simulink model "lab1_without_fuzzy_001"  (R2016a)
settings: Solver=ode45  StartTime=0.0  StopTime=10  RelTol=1e-3
values from neighbouring files (symbols this model uses):
  FORCE_Range_1 = -150    [fuzzy_controller_3_trimf_params.m]    (also in fuzzy_controller_5_gauss_params.m; fuzzy_controller_5_gbell_params.m; fuzzy_controller_5_trimf_optimal_params.m; fuzzy_controller_5_trimf_params.m)
  FORCE_Range_2 = 150    [fuzzy_controller_3_trimf_params.m]    (also in fuzzy_controller_5_gauss_params.m; fuzzy_controller_5_gbell_params.m; fuzzy_controller_5_trimf_optimal_params.m; fuzzy_controller_5_trimf_params.m)
  g = 9.81    [Variables_001.m]
  Kd = 141    [Variables_001.m]
  Kp = 1108    [Variables_001.m]
  l = 1    [Variables_001.m]
  M = 10    [Variables_001.m]
  m = 1    [Variables_001.m]
  q0 = 0.1    [Variables_001.m]
  taum = 0.001    [Variables_001.m]
undefined symbols (not defined in the file): fi_1_a, fi_1_b, fi_1_c, fi_1_d, fi_2_a, fi_2_b, fi_2_c, fi_3_a, fi_3_b, fi_3_c, fi_4_a, fi_4_b, fi_4_c, fi_5_a, fi_5_b, fi_5_c, fi_5_d, FORCE_1_a, FORCE_1_b, FORCE_1_c, FORCE_2_a, FORCE_2_b, FORCE_2_c, FORCE_3_a, FORCE_3_b, FORCE_3_c, FORCE_4_a, FORCE_4_b, FORCE_4_c, FORCE_5_a, FORCE_5_b, FORCE_5_c, omega_1_a, omega_1_b, omega_1_c, omega_1_d, omega_2_a, omega_2_b, omega_2_c, omega_3_a, omega_3_b, omega_3_c, omega_4_a, omega_4_b, omega_4_c, omega_5_a, omega_5_b, omega_5_c, omega_5_d
libraries: fuzblock x41, fuzwiz x2
(part 2 of 2)

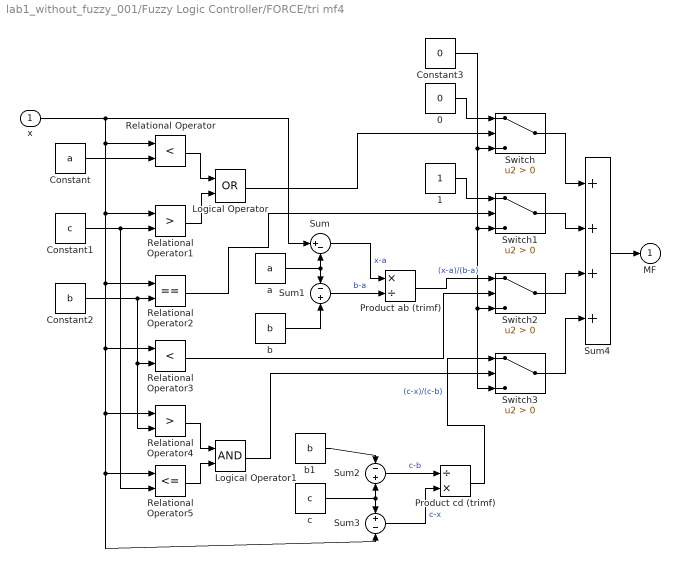
== system lab1_without_fuzzy_001/Fuzzy Logic Controller/FORCE/tri mf4 ==
  x : Inport
  0 : Constant  Value=0
  1 : Constant
  Constant : Constant  Value=a
  Constant1 : Constant  Value=c
  Constant2 : Constant  Value=b
  Constant3 : Constant  Value=0
  Logical Operator : Logic  Operator=OR  AllPortsSameDT=off  OutDataTypeStr=boolean
  Logical Operator1 : Logic  AllPortsSameDT=off  OutDataTypeStr=boolean
  Product ab (trimf) : Product  Inputs=*/  SaturateOnIntegerOverflow=on  InputSameDT=on  OutDataTypeStr=Inherit: Same as first input
  Product cd (trimf) : Product  Inputs=/*  SaturateOnIntegerOverflow=on  InputSameDT=on  OutDataTypeStr=Inherit: Same as first input
  Relational Operator : RelationalOperator  Operator=<  OutDataTypeStr=boolean
  Relational Operator1 : RelationalOperator  Operator=>  OutDataTypeStr=boolean
  Relational Operator2 : RelationalOperator  Operator===  OutDataTypeStr=boolean
  Relational Operator3 : RelationalOperator  Operator=<  OutDataTypeStr=boolean
  Relational Operator4 : RelationalOperator  Operator=>  OutDataTypeStr=boolean
  Relational Operator5 : RelationalOperator  Operator=<=  OutDataTypeStr=boolean
  Sum : Sum  Inputs=|+-  SaturateOnIntegerOverflow=on  InputSameDT=on  OutDataTypeStr=Inherit: Same as first input
  Sum1 : Sum  Inputs=-+  SaturateOnIntegerOverflow=on  InputSameDT=on  OutDataTypeStr=Inherit: Same as first input
  Sum2 : Sum  Inputs=-+  SaturateOnIntegerOverflow=on  InputSameDT=on  OutDataTypeStr=Inherit: Same as first input
  Sum3 : Sum  Inputs=+-  SaturateOnIntegerOverflow=on  InputSameDT=on  OutDataTypeStr=Inherit: Same as first input
  Sum4 : Sum  Inputs=++++
  Switch{,1..3} (4 alike) : Switch  Criteria=u2 > Threshold
  a : Constant  Value=a
  b : Constant  Value=b
  b1 : Constant  Value=b
  c : Constant  Value=c
  MF : Outport
  wires:
  0/1 -> Switch/1
  1/1 -> Switch1/1
  Constant/1 -> Relational Operator/2
  Relational Operator/1 -> Logical Operator/1
  Constant1/1 -> Relational Operator5/2, Relational Operator1/2
  Relational Operator1/1 -> Logical Operator/2
  Product ab (trimf)/1 -> Switch2/1  "(x-a)/(b-a)"
  a/1 -> Sum/2, Sum1/1
  b/1 -> Sum1/2
  Sum/1 -> Product ab (trimf)/1  "x-a"
  Sum1/1 -> Product ab (trimf)/2  "b-a"
  b1/1 -> Sum2/1
  x/1 -> Sum/1, Sum3/2, Relational Operator5/1, Relational Operator4/1, Relational Operator3/1, Relational Operator2/1, Relational Operator1/1, Relational Operator/1
  c/1 -> Sum3/1, Sum2/2
  Sum3/1 -> Product cd (trimf)/2  "c-x"
  Sum2/1 -> Product cd (trimf)/1  "c-b"
  Product cd (trimf)/1 -> Switch3/1  "(c-x)/(c-b)"
  Constant2/1 -> Relational Operator2/2, Relational Operator3/2, Relational Operator4/2
  Relational Operator4/1 -> Logical Operator1/1
  Relational Operator5/1 -> Logical Operator1/2
  Switch/1 -> Sum4/1
  Switch1/1 -> Sum4/2
  Switch2/1 -> Sum4/3
  Switch3/1 -> Sum4/4
  Constant3/1 -> Switch3/3, Switch2/3, Switch1/3, Switch/3
  Logical Operator1/1 -> Switch3/2
  Relational Operator3/1 -> Switch2/2
  Relational Operator2/1 -> Switch1/2
  Logical Operator/1 -> Switch/2
  Sum4/1 -> MF/1

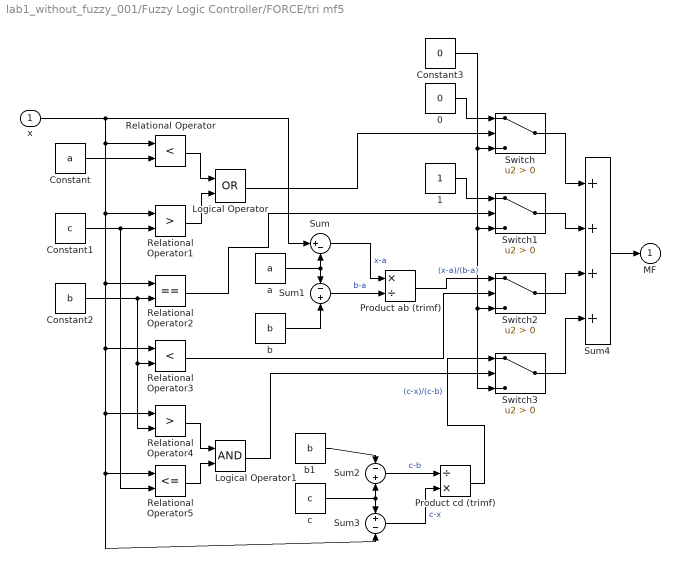
== system lab1_without_fuzzy_001/Fuzzy Logic Controller/FORCE/tri mf5 ==
  x : Inport
  0 : Constant  Value=0
  1 : Constant
  Constant : Constant  Value=a
  Constant1 : Constant  Value=c
  Constant2 : Constant  Value=b
  Constant3 : Constant  Value=0
  Logical Operator : Logic  Operator=OR  AllPortsSameDT=off  OutDataTypeStr=boolean
  Logical Operator1 : Logic  AllPortsSameDT=off  OutDataTypeStr=boolean
  Product ab (trimf) : Product  Inputs=*/  SaturateOnIntegerOverflow=on  InputSameDT=on  OutDataTypeStr=Inherit: Same as first input
  Product cd (trimf) : Product  Inputs=/*  SaturateOnIntegerOverflow=on  InputSameDT=on  OutDataTypeStr=Inherit: Same as first input
  Relational Operator : RelationalOperator  Operator=<  OutDataTypeStr=boolean
  Relational Operator1 : RelationalOperator  Operator=>  OutDataTypeStr=boolean
  Relational Operator2 : RelationalOperator  Operator===  OutDataTypeStr=boolean
  Relational Operator3 : RelationalOperator  Operator=<  OutDataTypeStr=boolean
  Relational Operator4 : RelationalOperator  Operator=>  OutDataTypeStr=boolean
  Relational Operator5 : RelationalOperator  Operator=<=  OutDataTypeStr=boolean
  Sum : Sum  Inputs=|+-  SaturateOnIntegerOverflow=on  InputSameDT=on  OutDataTypeStr=Inherit: Same as first input
  Sum1 : Sum  Inputs=-+  SaturateOnIntegerOverflow=on  InputSameDT=on  OutDataTypeStr=Inherit: Same as first input
  Sum2 : Sum  Inputs=-+  SaturateOnIntegerOverflow=on  InputSameDT=on  OutDataTypeStr=Inherit: Same as first input
  Sum3 : Sum  Inputs=+-  SaturateOnIntegerOverflow=on  InputSameDT=on  OutDataTypeStr=Inherit: Same as first input
  Sum4 : Sum  Inputs=++++
  Switch{,1..3} (4 alike) : Switch  Criteria=u2 > Threshold
  a : Constant  Value=a
  b : Constant  Value=b
  b1 : Constant  Value=b
  c : Constant  Value=c
  MF : Outport
  wires:
  0/1 -> Switch/1
  1/1 -> Switch1/1
  Constant/1 -> Relational Operator/2
  Relational Operator/1 -> Logical Operator/1
  Constant1/1 -> Relational Operator5/2, Relational Operator1/2
  Relational Operator1/1 -> Logical Operator/2
  Product ab (trimf)/1 -> Switch2/1  "(x-a)/(b-a)"
  a/1 -> Sum/2, Sum1/1
  b/1 -> Sum1/2
  Sum/1 -> Product ab (trimf)/1  "x-a"
  Sum1/1 -> Product ab (trimf)/2  "b-a"
  b1/1 -> Sum2/1
  x/1 -> Sum/1, Sum3/2, Relational Operator5/1, Relational Operator4/1, Relational Operator3/1, Relational Operator2/1, Relational Operator1/1, Relational Operator/1
  c/1 -> Sum3/1, Sum2/2
  Sum3/1 -> Product cd (trimf)/2  "c-x"
  Sum2/1 -> Product cd (trimf)/1  "c-b"
  Product cd (trimf)/1 -> Switch3/1  "(c-x)/(c-b)"
  Constant2/1 -> Relational Operator2/2, Relational Operator3/2, Relational Operator4/2
  Relational Operator4/1 -> Logical Operator1/1
  Relational Operator5/1 -> Logical Operator1/2
  Switch/1 -> Sum4/1
  Switch1/1 -> Sum4/2
  Switch2/1 -> Sum4/3
  Switch3/1 -> Sum4/4
  Constant3/1 -> Switch3/3, Switch2/3, Switch1/3, Switch/3
  Logical Operator1/1 -> Switch3/2
  Relational Operator3/1 -> Switch2/2
  Relational Operator2/1 -> Switch1/2
  Logical Operator/1 -> Switch/2
  Sum4/1 -> MF/1

== system lab1_without_fuzzy_001/Fuzzy Logic Controller/fi/trap mf1 ==
  x : Inport
  If Action Subsystem : fuzblock/Membership  Functions/Triangular MF/If Action Subsystem
  If Action Subsystem1 : fuzblock/Membership  Functions/Triangular MF/If Action Subsystem1
  If Action Subsystem2 : fuzblock/Membership  Functions/Trapezoidal MF/If Action Subsystem1
  If Action Subsystem8 : fuzblock/Membership  Functions/Trapezoidal MF/If Action Subsystem3
  If2 : If  IfExpression=(u1 < a) | (u1>d)  ElseIfExpressions=(u1 >= b) & (u1 <= c), u1 < b  ZeroCross=off
  Merge : Merge  Inputs=4
  MF : Outport
  wires:
  If Action Subsystem2/1 -> Merge/3
  If2/3 -> If Action Subsystem2/Action
  If Action Subsystem8/1 -> Merge/4
  If2/4 -> If Action Subsystem8/Action
  If Action Subsystem1/1 -> Merge/2
  If2/2 -> If Action Subsystem1/Action
  If Action Subsystem/1 -> Merge/1
  Merge/1 -> MF/1
  If2/1 -> If Action Subsystem/Action
  x/1 -> If Action Subsystem2/1, If Action Subsystem8/1, If2/1

== system lab1_without_fuzzy_001/Fuzzy Logic Controller/fi/trap mf5 ==
  x : Inport
  If Action Subsystem : fuzblock/Membership  Functions/Triangular MF/If Action Subsystem
  If Action Subsystem1 : fuzblock/Membership  Functions/Triangular MF/If Action Subsystem1
  If Action Subsystem2 : fuzblock/Membership  Functions/Trapezoidal MF/If Action Subsystem1
  If Action Subsystem8 : fuzblock/Membership  Functions/Trapezoidal MF/If Action Subsystem3
  If2 : If  IfExpression=(u1 < a) | (u1>d)  ElseIfExpressions=(u1 >= b) & (u1 <= c), u1 < b  ZeroCross=off
  Merge : Merge  Inputs=4
  MF : Outport
  wires:
  If Action Subsystem2/1 -> Merge/3
  If2/3 -> If Action Subsystem2/Action
  If Action Subsystem8/1 -> Merge/4
  If2/4 -> If Action Subsystem8/Action
  If Action Subsystem1/1 -> Merge/2
  If2/2 -> If Action Subsystem1/Action
  If Action Subsystem/1 -> Merge/1
  Merge/1 -> MF/1
  If2/1 -> If Action Subsystem/Action
  x/1 -> If Action Subsystem2/1, If Action Subsystem8/1, If2/1

== system lab1_without_fuzzy_001/Fuzzy Logic Controller/fi/tri mf2 ==
  x : Inport
  If : If  IfExpression=(u1<a) | (u1>c)  ElseIfExpressions=u1==b, u1 < b  ZeroCross=off
  If Action Subsystem : fuzblock/Membership  Functions/Triangular MF/If Action Subsystem
  If Action Subsystem1 : fuzblock/Membership  Functions/Triangular MF/If Action Subsystem1
  If Action Subsystem2 : fuzblock/Membership  Functions/Triangular MF/If Action Subsystem2
  If Action Subsystem3 : fuzblock/Membership  Functions/Triangular MF/If Action Subsystem3
  Merge : Merge  Inputs=4
  MF : Outport
  wires:
  If Action Subsystem3/1 -> Merge/3
  If/3 -> If Action Subsystem3/Action
  If Action Subsystem2/1 -> Merge/4
  If/4 -> If Action Subsystem2/Action
  If Action Subsystem1/1 -> Merge/2
  If/2 -> If Action Subsystem1/Action
  If Action Subsystem/1 -> Merge/1
  Merge/1 -> MF/1
  If/1 -> If Action Subsystem/Action
  x/1 -> If Action Subsystem3/1, If Action Subsystem2/1, If/1

== system lab1_without_fuzzy_001/Fuzzy Logic Controller/fi/tri mf3 ==
  x : Inport
  If : If  IfExpression=(u1<a) | (u1>c)  ElseIfExpressions=u1==b, u1 < b  ZeroCross=off
  If Action Subsystem : fuzblock/Membership  Functions/Triangular MF/If Action Subsystem
  If Action Subsystem1 : fuzblock/Membership  Functions/Triangular MF/If Action Subsystem1
  If Action Subsystem2 : fuzblock/Membership  Functions/Triangular MF/If Action Subsystem2
  If Action Subsystem3 : fuzblock/Membership  Functions/Triangular MF/If Action Subsystem3
  Merge : Merge  Inputs=4
  MF : Outport
  wires:
  If Action Subsystem3/1 -> Merge/3
  If/3 -> If Action Subsystem3/Action
  If Action Subsystem2/1 -> Merge/4
  If/4 -> If Action Subsystem2/Action
  If Action Subsystem1/1 -> Merge/2
  If/2 -> If Action Subsystem1/Action
  If Action Subsystem/1 -> Merge/1
  Merge/1 -> MF/1
  If/1 -> If Action Subsystem/Action
  x/1 -> If Action Subsystem3/1, If Action Subsystem2/1, If/1

== system lab1_without_fuzzy_001/Fuzzy Logic Controller/fi/tri mf4 ==
  x : Inport
  If : If  IfExpression=(u1<a) | (u1>c)  ElseIfExpressions=u1==b, u1 < b  ZeroCross=off
  If Action Subsystem : fuzblock/Membership  Functions/Triangular MF/If Action Subsystem
  If Action Subsystem1 : fuzblock/Membership  Functions/Triangular MF/If Action Subsystem1
  If Action Subsystem2 : fuzblock/Membership  Functions/Triangular MF/If Action Subsystem2
  If Action Subsystem3 : fuzblock/Membership  Functions/Triangular MF/If Action Subsystem3
  Merge : Merge  Inputs=4
  MF : Outport
  wires:
  If Action Subsystem3/1 -> Merge/3
  If/3 -> If Action Subsystem3/Action
  If Action Subsystem2/1 -> Merge/4
  If/4 -> If Action Subsystem2/Action
  If Action Subsystem1/1 -> Merge/2
  If/2 -> If Action Subsystem1/Action
  If Action Subsystem/1 -> Merge/1
  Merge/1 -> MF/1
  If/1 -> If Action Subsystem/Action
  x/1 -> If Action Subsystem3/1, If Action Subsystem2/1, If/1

== system lab1_without_fuzzy_001/Fuzzy Logic Controller/omega/trap mf1 ==
  x : Inport
  If Action Subsystem : fuzblock/Membership  Functions/Triangular MF/If Action Subsystem
  If Action Subsystem1 : fuzblock/Membership  Functions/Triangular MF/If Action Subsystem1
  If Action Subsystem2 : fuzblock/Membership  Functions/Trapezoidal MF/If Action Subsystem1
  If Action Subsystem8 : fuzblock/Membership  Functions/Trapezoidal MF/If Action Subsystem3
  If2 : If  IfExpression=(u1 < a) | (u1>d)  ElseIfExpressions=(u1 >= b) & (u1 <= c), u1 < b  ZeroCross=off
  Merge : Merge  Inputs=4
  MF : Outport
  wires:
  If Action Subsystem2/1 -> Merge/3
  If2/3 -> If Action Subsystem2/Action
  If Action Subsystem8/1 -> Merge/4
  If2/4 -> If Action Subsystem8/Action
  If Action Subsystem1/1 -> Merge/2
  If2/2 -> If Action Subsystem1/Action
  If Action Subsystem/1 -> Merge/1
  Merge/1 -> MF/1
  If2/1 -> If Action Subsystem/Action
  x/1 -> If Action Subsystem2/1, If Action Subsystem8/1, If2/1

== system lab1_without_fuzzy_001/Fuzzy Logic Controller/omega/trap mf5 ==
  x : Inport
  If Action Subsystem : fuzblock/Membership  Functions/Triangular MF/If Action Subsystem
  If Action Subsystem1 : fuzblock/Membership  Functions/Triangular MF/If Action Subsystem1
  If Action Subsystem2 : fuzblock/Membership  Functions/Trapezoidal MF/If Action Subsystem1
  If Action Subsystem8 : fuzblock/Membership  Functions/Trapezoidal MF/If Action Subsystem3
  If2 : If  IfExpression=(u1 < a) | (u1>d)  ElseIfExpressions=(u1 >= b) & (u1 <= c), u1 < b  ZeroCross=off
  Merge : Merge  Inputs=4
  MF : Outport
  wires:
  If Action Subsystem2/1 -> Merge/3
  If2/3 -> If Action Subsystem2/Action
  If Action Subsystem8/1 -> Merge/4
  If2/4 -> If Action Subsystem8/Action
  If Action Subsystem1/1 -> Merge/2
  If2/2 -> If Action Subsystem1/Action
  If Action Subsystem/1 -> Merge/1
  Merge/1 -> MF/1
  If2/1 -> If Action Subsystem/Action
  x/1 -> If Action Subsystem2/1, If Action Subsystem8/1, If2/1

== system lab1_without_fuzzy_001/Fuzzy Logic Controller/omega/tri mf2 ==
  x : Inport
  If : If  IfExpression=(u1<a) | (u1>c)  ElseIfExpressions=u1==b, u1 < b  ZeroCross=off
  If Action Subsystem : fuzblock/Membership  Functions/Triangular MF/If Action Subsystem
  If Action Subsystem1 : fuzblock/Membership  Functions/Triangular MF/If Action Subsystem1
  If Action Subsystem2 : fuzblock/Membership  Functions/Triangular MF/If Action Subsystem2
  If Action Subsystem3 : fuzblock/Membership  Functions/Triangular MF/If Action Subsystem3
  Merge : Merge  Inputs=4
  MF : Outport
  wires:
  If Action Subsystem3/1 -> Merge/3
  If/3 -> If Action Subsystem3/Action
  If Action Subsystem2/1 -> Merge/4
  If/4 -> If Action Subsystem2/Action
  If Action Subsystem1/1 -> Merge/2
  If/2 -> If Action Subsystem1/Action
  If Action Subsystem/1 -> Merge/1
  Merge/1 -> MF/1
  If/1 -> If Action Subsystem/Action
  x/1 -> If Action Subsystem3/1, If Action Subsystem2/1, If/1

== system lab1_without_fuzzy_001/Fuzzy Logic Controller/omega/tri mf3 ==
  x : Inport
  If : If  IfExpression=(u1<a) | (u1>c)  ElseIfExpressions=u1==b, u1 < b  ZeroCross=off
  If Action Subsystem : fuzblock/Membership  Functions/Triangular MF/If Action Subsystem
  If Action Subsystem1 : fuzblock/Membership  Functions/Triangular MF/If Action Subsystem1
  If Action Subsystem2 : fuzblock/Membership  Functions/Triangular MF/If Action Subsystem2
  If Action Subsystem3 : fuzblock/Membership  Functions/Triangular MF/If Action Subsystem3
  Merge : Merge  Inputs=4
  MF : Outport
  wires:
  If Action Subsystem3/1 -> Merge/3
  If/3 -> If Action Subsystem3/Action
  If Action Subsystem2/1 -> Merge/4
  If/4 -> If Action Subsystem2/Action
  If Action Subsystem1/1 -> Merge/2
  If/2 -> If Action Subsystem1/Action
  If Action Subsystem/1 -> Merge/1
  Merge/1 -> MF/1
  If/1 -> If Action Subsystem/Action
  x/1 -> If Action Subsystem3/1, If Action Subsystem2/1, If/1

== system lab1_without_fuzzy_001/Fuzzy Logic Controller/omega/tri mf4 ==
  x : Inport
  If : If  IfExpression=(u1<a) | (u1>c)  ElseIfExpressions=u1==b, u1 < b  ZeroCross=off
  If Action Subsystem : fuzblock/Membership  Functions/Triangular MF/If Action Subsystem
  If Action Subsystem1 : fuzblock/Membership  Functions/Triangular MF/If Action Subsystem1
  If Action Subsystem2 : fuzblock/Membership  Functions/Triangular MF/If Action Subsystem2
  If Action Subsystem3 : fuzblock/Membership  Functions/Triangular MF/If Action Subsystem3
  Merge : Merge  Inputs=4
  MF : Outport
  wires:
  If Action Subsystem3/1 -> Merge/3
  If/3 -> If Action Subsystem3/Action
  If Action Subsystem2/1 -> Merge/4
  If/4 -> If Action Subsystem2/Action
  If Action Subsystem1/1 -> Merge/2
  If/2 -> If Action Subsystem1/Action
  If Action Subsystem/1 -> Merge/1
  Merge/1 -> MF/1
  If/1 -> If Action Subsystem/Action
  x/1 -> If Action Subsystem3/1, If Action Subsystem2/1, If/1
